simulink model "model"  (R2020a)
settings: Solver=VariableStepAuto  StartTime=0.0  StopTime=.3  MaxStep=1e-6  RelTol=1e-3  EnableMultiTasking=on
values from neighbouring files (symbols this model uses):
  f = 20    [data_collection.m]
  g = A(q,8)    [data_collection.m]
  g0 = 14e-6    (= 1.4e-05)    [data_collection.m]
  lf = 400e-6    (= 0.0004)    [data_collection.m]
  m = 2.0933e-6    (= 2.0933e-06)    [data_collection.m]
  tfd = 25e-6    (= 2.5e-05)    [data_collection.m]
  tp = 120e-9    (= 1.2e-07)    [data_collection.m]
  wb = 30e-6    (= 3e-05)    [data_collection.m]
  wt = 9e-6    (= 9e-06)    [data_collection.m]
libraries: simulink x1
settings Model: SimulationMode=accelerator  Creator=OXAALJ  LastModifiedBy=galarm2
settings SolverCC: MaxOrder=2  MaxConsecutiveZCs=10  MaxConsecutiveMinStep=10  ZeroCrossControl=DisableAll
settings DataIOCC: LimitDataPoints=on  SaveFormat=Array  DSMLogging=off  ReturnWorkspaceOutputs=off
settings OptimizationCC: EfficientMapNaN2IntZero=off  LifeSpan=inf
settings DebuggingCC: UnderspecifiedInitializationDetection=Classic  MergeDetectMultiDrivingBlocksExec=none  SolverPrmCheckMsg=warning  MultiTaskDSMMsg=warning  MultiTaskCondExecSysMsg=none  StateNameClashWarn=warning  SFUnexpectedBacktrackingDiag=warning  SFNoUnconditionalDefaultTransitionDiag=warning  SFExecutionAtInitializationDiag=none  ArithmeticOperatorsInVariantConditions=warning
settings HardwareCC: ProdBitPerPointer=32  ProdBitPerSizeT=32  ProdBitPerPtrDiffT=32  ProdLargestAtomicFloat=None  ProdIntDivRoundTo=Undefined  ProdEndianess=Unspecified  ProdWordSize=32  ProdHWDeviceType=32-bit Generic  TargetBitPerPointer=64  TargetBitPerSizeT=64  TargetBitPerPtrDiffT=64  TargetLongLongMode=on  TargetIntDivRoundTo=Zero  TargetEndianess=LittleEndian  TargetWordSize=64  TargetHWDeviceType=MATLAB Host  ProdEqTarget=off
settings ModelReferenceCC: PropagateSignalLabelsOutOfModel=off
settings SFSimCC: SimUseLocalCustomCode=off  CustomCodeUndefinedFunction=UseInterfaceOnly
settings CodeAppCC: MaxIdLength=128
settings GRTTargetCC: TargetLangStandard=C89/C90 (ANSI)  CombineOutputUpdateFcns=off  GRTInterface=on
settings ConfigComp: CovMetricSettings=dw  CovHtmlReporting=on  CovSaveCumulativeToWorkspaceVar=on  CovSaveSingleToWorkspaceVar=on  CovExternalEMLEnable=off  CovSFcnEnable=off

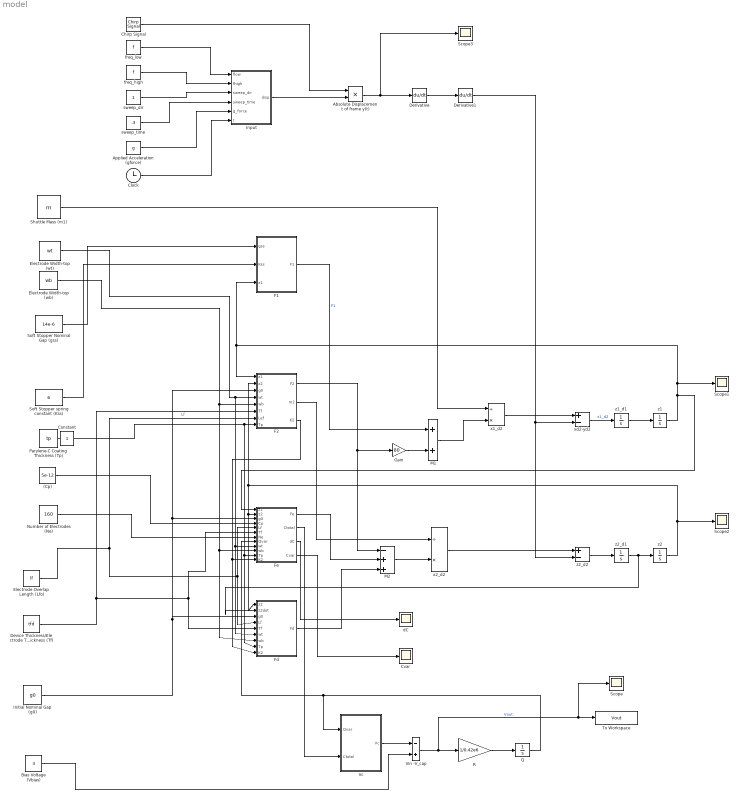
== system model ==
  " M2" : Sum  Inputs=-++  RndMeth=Nearest
  (Cp) : Constant  Value=5e-12  VectorParams1D=off
  Absolute Displacement of frame y(t) : Product
  Applied Acceleration (gforce) : Constant  Value=g
  Bias Voltage (Vbias) : Constant  Value=3
  Chirp Signal : simulink/Sources/Chirp Signal  f1=f  T=0.3  f2=f
  Clock : Clock
  Cvar : Scope
  Derivative : Derivative
  Derivative1 : Derivative
  Device Thickness/Electrode Thickness (Tf) : Constant  Value=tfd
  Electrode Overlap Length (Lfo) : Constant  Value=lf
  Electrode Width-top (wb) : Constant  Value=wb
  Electrode Width-top (wt) : Constant  Value=wt
  F1 : MATLAB Function  TreatAsAtomicUnit=on
  F2 : MATLAB Function  TreatAsAtomicUnit=on
  Fd : MATLAB Function  TreatAsAtomicUnit=on
  Fe : MATLAB Function  TreatAsAtomicUnit=on
  Gain : Gain  Gain=80
  Initial Nominal Gap (g0) : Constant  Value=g0
  Input : MATLAB Function  TreatAsAtomicUnit=on
  M1 : Sum  RndMeth=Nearest
  Number of Electrodes (Ne) : Constant  Value=160
  Parylene-C Coating Thickness (Tp) : Constant  Value=tp
  Q : Integrator
  R : Gain  Gain=1/0.42e6
  Scope{,1..3} (4 alike) : Scope
  Shuttle Mass (m1) : Constant  Value=m
  Soft Stopper Nominal Gap (gss) : Constant  Value=14e-6
  Soft Stopper spring constant (Kss) : Constant  Value=6
  To Workspace : ToWorkspace  VariableName=Vout  SampleTime=-1
      settings: Save2DSignal=2-D array (concatenate along first dimension)
  Vc : MATLAB Function  TreatAsAtomicUnit=on
  Vin -V_cap : Sum  Inputs=-+  RndMeth=Nearest
  dC : Scope
  freq_high : Constant  Value=f
  freq_low : Constant  Value=f
  sweep_dir : Constant
  sweep_time : Constant  Value=.3
  x1_d2 : Product  Inputs=/*
  x2_d2 : Product  Inputs=/*
  xd2-yd2 : Sum  Inputs=+-  RndMeth=Nearest
  z1 : Integrator
  z1_d1 : Integrator
  z2 : Integrator
  z2_d1 : Integrator
  z2_d2 : Sum  Inputs=+-  RndMeth=Nearest
  Constant : Constant  IOType=siggen
  wires:
  F1/1(F1) -> M1/1  "F1"
  Shuttle Mass (m1)/1 -> x1_d2/1
  Initial Nominal Gap (g0)/1 -> F2/3(g0), Fe/3(g0), Fd/3(g0)
  Bias Voltage (Vbias)/1 -> Vin -V_cap/2
  Vin -V_cap/1 -> Scope/1, To Workspace/1, R/1  "Vout"
  R/1 -> Q/1
  Q/1 -> Fe/8(Qvar), Vc/1(Qvar)
  Electrode Overlap Length (Lfo)/1 -> F2/7(Lef), Fd/4(Lf), Fe/5(Lf)  "Lf"
  (Cp)/1 -> Fe/4(Cp)
  Device Thickness/Electrode Thickness (Tf)/1 -> F2/6(Tf), Fd/5(Tf), Fe/6(Tf)
  Soft Stopper spring constant (Kss)/1 -> F1/2(Kss)
  M1/1 -> x1_d2/2
  x1_d2/1 -> xd2-yd2/1
  xd2-yd2/1 -> z1_d1/1  "z1_d2"
  z1_d1/1 -> z1/1
  x2_d2/1 -> z2_d2/1
  z2_d1/1 -> Fd/2(z2dot), z2/1
  z2/1 -> Scope2/1, Fd/1(z2), Fe/2(z2), F2/2(z2)
  " M2"/1 -> x2_d2/2
  Soft Stopper Nominal Gap (gss)/1 -> F1/1(gss)
  Input/1(disp) -> Absolute Displacement of frame y(t)/2
  freq_high/1 -> Input/2(fhigh)
  Applied Acceleration (gforce)/1 -> Input/5(g_force)
  Clock/1 -> Input/6(t)
  F2/1(F2) -> Gain/1, " M2"/1
  F2/2(m2) -> x2_d2/1
  Parylene-C Coating Thickness (Tp)/1 -> Fd/8(Tp), Fe/11(Tp), F2/8(Tp)
  Fe/1(Fe) -> " M2"/2
  Fe/2(Ctotal) -> Vc/2(Ctotal)
  Fd/1(Fd) -> " M2"/3
  Vc/1(Vc) -> Vin -V_cap/1
  Electrode Width-top (wt)/1 -> Fd/6(wt), Fe/9(wt), F2/4(wt)
  Electrode Width-top (wb)/1 -> Fd/7(wb), Fe/10(wb), F2/5(wb)
  Absolute Displacement of frame y(t)/1 -> Scope3/1, Derivative/1
  Derivative/1 -> Derivative1/1
  freq_low/1 -> Input/1(flow)
  sweep_time/1 -> Input/4(sweep_time)
  sweep_dir/1 -> Input/3(sweep_dir)
  z2_d2/1 -> z2_d1/1
  Derivative1/1 -> z2_d2/2, xd2-yd2/2
  Gain/1 -> M1/2
  z1/1 -> Scope1/1, F2/1(z1), F1/3(z1), Fe/1(z1)
  Number of Electrodes (Ne)/1 -> Fe/7(Ne)
  Fe/3(dC) -> dC/1
  Fe/4(Cvar) -> Cvar/1
  F2/3(K2) -> Fd/9(K2), Fe/12(K2)
  Chirp Signal/1 -> Absolute Displacement of frame y(t)/1

== matlab function model/F1 ==
  data: gss input; Kss input; z1 input; F1 output
function F1 = fcn(gss,Kss,z1)
% This function calculates the force F1
% Device Parameters

% Meg Value
k1 = 0.16;
Fsp = (-k1.*z1); % suspension beam force

% Fss
if abs(z1) < gss
    Fss = 0; % stopper not engaged
else
    Fss = Kss*(abs(z1)-gss)*sign(z1); % stopper is engaged
end

F1 = Fss + Fsp;
end

== matlab function model/Fd ==
  data: z2 input; z2dot input; g0 input; Fd output; Lf input; Tf input; wt input; wb input; Tp input; K2 input
function Fd = fcn(z2,z2dot,g0,Lf,Tf,wt,wb,Tp,K2)
% This function calculates the force F2
% Device Parameters
gp = g0 - 2*Tp; % minimum air gap 
eta = 1.849e-5; % Dynamic viscosity of air (kg/m*s)
% ws = mean([wt,wb]); % Avg. Electrode width
% I = (1/12)*Tf*(ws^3); % Moment of Inertia average width
% E = 180e9; % The Young's modulous 

% Scaling term for Damping force
scale = 0.015;
% set = 0;
% if abs(z2) >= gp
%     set = set + 1;
% end
% 
% if set < 1
%     scale = 0.015; % Scaling term for Damping force
% else
%     scale = 0.01965; 
% end

% Tilt angle
a = (wb-wt)/Lf; % previous calculation
% a = ((wb-wt)/Lf)-(((K2*(abs(z2)-gp))*(Lf^2))/(3*E*I)); % new calculation

% Fd_l
ul  =  gp + z2; % Left-hand side ho
ll  =  ul + a*Lf; % Left-hand side hl
A1_l  =  -ul*Lf/(ul + 2*a)* z2dot; % The c1 parameter, left
A2_l  =  12*eta*a^-2/(2*ul + a*Lf) * z2dot; % The c1 parameter, left
Fd_l   =  Tf*(Lf*A2_l - 6*eta*Lf/a/ul/ll*A1_l + 6*eta*Lf*a^-4/ll*z2dot + 12*eta*a^-3 * z2dot * (log(abs(ul./ll))) );

% Fd_r
ur  =  gp - z2;  
lr  =  ur + a*Lf;
A1_r  =  -ur*Lf/(ur + 2*a)* z2dot; % The c1 parameter, right
A2_r  =  12*eta*a^-2/(2*ur + a*Lf) * z2dot; % The c1 parameter, right
Fd_r   =  Tf*(Lf*A2_r - 6*eta*Lf/a/ur/lr*A1_r + 6*eta*Lf*a^-4/lr*z2dot - 12*eta*a^-3 * z2dot * (log(abs(ur./lr))) );

% Fd
Fd  =  -scale*(Fd_l + Fd_r);
end

== matlab function model/Vc ==
  data: Qvar input; Vc output; Ctotal input
function Vc = fcn(Qvar,Ctotal)
% This function calculates the Vc value
Vc = Qvar/Ctotal;
end

== matlab function model/Fe ==
  data: z1 input; z2 input; g0 input; Cp input; Fe output; Lf input; Tf input; Ne input; Qvar input; wt input; wb input; Tp input; Ctotal output; dC output; Cvar output; K2 input
function [Fe,Ctotal,dC,Cvar] = fcn(z1,z2,g0,Cp,Lf,Tf,Ne,Qvar,wt,wb,Tp,K2)
% This function calculates the force F2
% Device Parameters
gp = g0 - 2*Tp; % minimum air gap 
ws = mean([wt,wb]); % Avg. Electrode width
I = (1/12)*Tf*(ws^3); % Moment of Inertia average width
E = 180e9; % The Young's modulous 
e = 8.85e-12; % Permittivity of free space
ep = 3.2; % Relative Permittivity of Parylene-C
scale = 1;
Cvar = 0;

% Tilt angle
a = (wb-wt)/Lf; % previous calculation
% a = ((wb-wt)/Lf)-(((K2*(abs(z2)-g0))*(Lf^2))/(3*E*I)); % new calculation

if abs(z2) < gp % The electrodes are not in contact
    % Cvar_r
    Crl = (ep.*e.*Lf.*Tf)/Tp;
    Cair_r = ((e.*Tf)/(2.*a)).*(log(((g0 - z2 + 2.*a.*Lf)./(g0 - z2))));
    Cvar_r = 1/((1/Crl)+(1/Cair_r)+(1/Crl));
    % Cvar_l
    Cair_l = ((e.*Tf)./(2.*a)).*(log(((g0 + z2 + 2.*a.*Lf)./(g0 + z2))));
    Cvar_l = 1./((1/Crl)+(1/Cair_l)+(1/Crl));
    % Cvar
    Cvar = (Cvar_r + Cvar_l).*(Ne/2);
elseif abs(z2) >= gp % The electrodes are in contact
    % Colliding Electrode
    Crl = (ep.*e.*Lf.*Tf)/Tp;
    % d = (wb-wt)-(((K2*(abs(z1)-abs(z2))*(Lf^3))/(3*E*I)));
    % d = (wb-wt)-(((K2*(abs(z1)-g0)*(Lf^3))/(3*E*I)));
    d = (wb-wt)-(((K2*(abs(z2)-g0))*(Lf^3))/(3*E*I));
    % Cair_c = ((e*Tf*(Lf^2))/(2*d))*(log(abs(d-2*Tp))-log(abs((2*Tp))));
    % Cair_c = ((e*Tf*Lf)/(d))*(log((2*d - 2*Tp)/(2*Tp)));
    Cair_c = ((e*Tf*Lf)/(d))*(log((2*Tp + 2*d)/(2*Tp)));
    Cvar_c = 1./((1/Crl)+(1/Cair_c)+(1/Crl));
    % Non-colliding Electrode
    Cair_nc = ((e.*Tf)./(2.*a)).*(log((g0 + abs(z2) + 2.*a.*Lf)./(g0 + abs(z2))));
    Cvar_nc = 1./((1/Crl)+(1/Cair_nc)+(1/Crl));
    % Cvar
    Cvar = (Cvar_nc + Cvar_c).*(Ne/2);     
end

% Ctotal
Ctotal = Cvar + Cp;

% dC is divided by four here because nf is total electrodes, not number of electrode pairs
dC = ((e*Ne*Tf)./(4.*a))*( ((2*z2)/(gp^2 - z2^2)) - ((2*z2)/((gp + 2*Lf*a)^2 - z2^2) ));
% dC = ((e*Ne*Lf)./(4.*a))*( ((2*z2)/(g0^2 - z2^2)) - ((2*z2)/((g0 + 2*Tf*a)^2 - z2^2) ));

% dC = (Ne*((2*((g0 + 2*wb - 2*wt - z2)/(g0 - z2)^2 - 1/(g0 - z2))*(g0 - z2)*(wb - wt))/(Lf*Tf*e*log((g0 + 2*wb - 2*wt - z2)/(g0 - z2))^2*((2*wb - 2*wt)/(Lf*Tf*e*log((g0 + 2*wb - 2*wt - z2)/(g0 - z2))) + (2*Tp)/(Lf*Tf*e*ep))^2*(g0 + 2*wb - 2*wt - z2)) + (2*(g0 + z2)*(wb - wt)*(1/(g0 + z2) - (g0 + 2*wb - 2*wt + z2)/(g0 + z2)^2))/(Lf*Tf*e*log((g0 + 2*wb - 2*wt + z2)/(g0 + z2))^2*((2*wb - 2*wt)/(Lf*Tf*e*log((g0 + 2*wb - 2*wt + z2)/(g0 + z2))) + (2*Tp)/(Lf*Tf*e*ep))^2*(g0 + 2*wb - 2*wt + z2))))/2;
% dC = (Ne*(((K2*Lf^2*sign(z2))/(3*E*I*Tf*e*log(((2*K2*(g0 - abs(z2))*Lf^3)/(3*E*I) + 2*Tp + 2*wb - 2*wt)/(2*Tp))) - (2*K2*Lf^2*sign(z2)*((K2*(g0 - abs(z2))*Lf^3)/(3*E*I) + wb - wt))/(3*E*I*Tf*e*log((2*Tp + 2*wb - 2*wt + (2*K2*Lf^3*(g0 - abs(z2)))/(3*E*I))/(2*Tp))^2*((2*K2*(g0 - abs(z2))*Lf^3)/(3*E*I) + 2*Tp + 2*wb - 2*wt)))/((wb - wt + (K2*Lf^3*(g0 - abs(z2)))/(3*E*I))/(Lf*Tf*e*log((2*Tp + 2*wb - 2*wt + (2*K2*Lf^3*(g0 - abs(z2)))/(3*E*I))/(2*Tp))) + (2*Tp)/(Lf*Tf*e*ep))^2 + (2*(sign(z2)/(g0 + abs(z2)) - (sign(z2)*(g0 + 2*wb - 2*wt + abs(z2)))/(g0 + abs(z2))^2)*(g0 + abs(z2))*(wb - wt))/(Lf*Tf*e*log((g0 + 2*wb - 2*wt + abs(z2))/(g0 + abs(z2)))^2*((2*wb - 2*wt)/(Lf*Tf*e*log((g0 + 2*wb - 2*wt + abs(z2))/(g0 + abs(z2)))) + (2*Tp)/(Lf*Tf*e*ep))^2*(g0 + 2*wb - 2*wt + abs(z2)))))/2;

% dC = 0;
% % For no collision
% if abs(z2) < gp % The electrodes are not in contact
%     % g0
%     dC = (Ne*((2*((g0 + 2*wb - 2*wt - z2)/(g0 - z2)^2 - 1/(g0 - z2))*(g0 - z2)*(wb - wt))/(Lf*Tf*e*log((g0 + 2*wb - 2*wt - z2)/(g0 - z2))^2*((2*wb - 2*wt)/(Lf*Tf*e*log((g0 + 2*wb - 2*wt - z2)/(g0 - z2))) + (2*Tp)/(Lf*Tf*e*ep))^2*(g0 + 2*wb - 2*wt - z2)) + (2*(g0 + z2)*(wb - wt)*(1/(g0 + z2) - (g0 + 2*wb - 2*wt + z2)/(g0 + z2)^2))/(Lf*Tf*e*log((g0 + 2*wb - 2*wt + z2)/(g0 + z2))^2*((2*wb - 2*wt)/(Lf*Tf*e*log((g0 + 2*wb - 2*wt + z2)/(g0 + z2))) + (2*Tp)/(Lf*Tf*e*ep))^2*(g0 + 2*wb - 2*wt + z2))))/2;
%     % gp
%     % dC = (Ne*((2*((gp + 2*wb - 2*wt - z2)/(gp - z2)^2 - 1/(gp - z2))*(gp - z2)*(wb - wt))/(Lf*Tf*e*log((gp + 2*wb - 2*wt - z2)/(gp - z2))^2*((2*wb - 2*wt)/(Lf*Tf*e*log((gp + 2*wb - 2*wt - z2)/(gp - z2))) + (2*Tp)/(Lf*Tf*e*ep))^2*(gp + 2*wb - 2*wt - z2)) + (2*(gp + z2)*(wb - wt)*(1/(gp + z2) - (gp + 2*wb - 2*wt + z2)/(gp + z2)^2))/(Lf*Tf*e*log((gp + 2*wb - 2*wt + z2)/(gp + z2))^2*((2*wb - 2*wt)/(Lf*Tf*e*log((gp + 2*wb - 2*wt + z2)/(gp + z2))) + (2*Tp)/(Lf*Tf*e*ep))^2*(gp + 2*wb - 2*wt + z2))))/2;
% % For collision
% elseif abs(z2) >= gp % The electrodes are in contact
%     % g0
%     dC = (Ne*(((K2*Lf^2*sign(z2))/(3*E*I*Tf*e*log(((2*K2*(g0 - abs(z2))*Lf^3)/(3*E*I) + 2*Tp + 2*wb - 2*wt)/(2*Tp))) - (2*K2*Lf^2*sign(z2)*((K2*(g0 - abs(z2))*Lf^3)/(3*E*I) + wb - wt))/(3*E*I*Tf*e*log((2*Tp + 2*wb - 2*wt + (2*K2*Lf^3*(g0 - abs(z2)))/(3*E*I))/(2*Tp))^2*((2*K2*(g0 - abs(z2))*Lf^3)/(3*E*I) + 2*Tp + 2*wb - 2*wt)))/((wb - wt + (K2*Lf^3*(g0 - abs(z2)))/(3*E*I))/(Lf*Tf*e*log((2*Tp + 2*wb - 2*wt + (2*K2*Lf^3*(g0 - abs(z2)))/(3*E*I))/(2*Tp))) + (2*Tp)/(Lf*Tf*e*ep))^2 + (2*(sign(z2)/(g0 + abs(z2)) - (sign(z2)*(g0 + 2*wb - 2*wt + abs(z2)))/(g0 + abs(z2))^2)*(g0 + abs(z2))*(wb - wt))/(Lf*Tf*e*log((g0 + 2*wb - 2*wt + abs(z2))/(g0 + abs(z2)))^2*((2*wb - 2*wt)/(Lf*Tf*e*log((g0 + 2*wb - 2*wt + abs(z2))/(g0 + abs(z2)))) + (2*Tp)/(Lf*Tf*e*ep))^2*(g0 + 2*wb - 2*wt + abs(z2)))))/2;
%     % gp
%     % dC = (Ne*(((K2*Lf^2*sign(z2))/(3*E*I*Tf*e*log(((2*K2*(gp - abs(z2))*Lf^3)/(3*E*I) + 2*Tp + 2*wb - 2*wt)/(2*Tp))) - (2*K2*Lf^2*sign(z2)*((K2*(gp - abs(z2))*Lf^3)/(3*E*I) + wb - wt))/(3*E*I*Tf*e*log((2*Tp + 2*wb - 2*wt + (2*K2*Lf^3*(gp - abs(z2)))/(3*E*I))/(2*Tp))^2*((2*K2*(gp - abs(z2))*Lf^3)/(3*E*I) + 2*Tp + 2*wb - 2*wt)))/((wb - wt + (K2*Lf^3*(gp - abs(z2)))/(3*E*I))/(Lf*Tf*e*log((2*Tp + 2*wb - 2*wt + (2*K2*Lf^3*(gp - abs(z2)))/(3*E*I))/(2*Tp))) + (2*Tp)/(Lf*Tf*e*ep))^2 + (2*(sign(z2)/(gp + abs(z2)) - (sign(z2)*(gp + 2*wb - 2*wt + abs(z2)))/(gp + abs(z2))^2)*(gp + abs(z2))*(wb - wt))/(Lf*Tf*e*log((gp + 2*wb - 2*wt + abs(z2))/(gp + abs(z2)))^2*((2*wb - 2*wt)/(Lf*Tf*e*log((gp + 2*wb - 2*wt + abs(z2))/(gp + abs(z2)))) + (2*Tp)/(Lf*Tf*e*ep))^2*(gp + 2*wb - 2*wt + abs(z2)))))/2;
% end

% Fe
NFe = -1*((Qvar^2)/(2*Ctotal^2))*dC;
Fe = NFe./(Ne/2)*scale;
end

== matlab function model/Input ==
  data: flow input; fhigh input; sweep_dir input; sweep_time input; g_force input; disp output; t input
function disp  = fcn(flow,fhigh,sweep_dir,sweep_time,g_force,t)
ramp = 200e-3;

if sweep_dir > 0
    %upsweep
    if t < ramp
        freq = (t/sweep_time)*(fhigh-flow) + flow;
        disp = (t/ramp)* (g_force/(4.0243*freq^2)); %const = (2*pi())^2/9.81
        % vel = (t/ramp)*(g_force*9.81)/(2*pi*freq);
    else
        freq = (t/sweep_time)*(fhigh-flow) + flow;
        disp = g_force/(4.0243*freq^2);   %const = (2*pi())^2/9.81
        % vel = (g_force*9.81)/(2*pi*freq);
        % disp = g/(4.0243*((fhigh-flow)/2)^2); 
        % freq = (0.5) * (fhigh+flow);
        % disp = g/(4.0243*freq^2);  %const = (2*pi())^2/9.81
    end
else
    %downsweep
    if t < ramp
        freq = fhigh - (t/sweep_time)*(fhigh-flow);
        disp = (t/ramp)* (g_force/(4.0243*freq^2)); %const = (2*pi())^2/9.81
        % vel = (t/ramp)*(g_force*9.81)/(2*pi*freq);
    else
        freq = fhigh - (t/sweep_time)*(fhigh-flow);
        disp = g_force/(4.0243*freq^2);  %const = (2*pi())^2/9.81
        % vel = (g_force*9.81)/(2*pi*freq);
        % disp = g/(4.0243*((fhigh-flow)/2)^2); 
        % freq = (0.5) * (fhigh+flow);
        % disp = g/(4.0243*freq^2);  %const = (2*pi())^2/9.81
    end
end
end

== matlab function model/F2 ==
  data: z1 input; z2 input; F2 output; g0 input; m2 output; wt input; wb input; Tf input; Lef input; Tp input; K2 output
function [F2,m2,K2] = fcn(z1,z2,g0,wt,wb,Tf,Lef,Tp)
% This function calculates the force F2
% Device Parameters
gp = g0 - 2*Tp; % minimum air gap
E = 180e9; % The Young's modulous 
rho = 2333; % density (kg/m3)
ws = mean([wt,wb]); % Avg. Electrode width
Lf = Lef + 50e-6; % Account for non-overlap
I = (1/12)*Tf*(ws^3); % Moment of Inertia average width
% h = (wb-wt)*(Lef/Lf); % height function
% I = (1/12)*Tf*(h^3); % Moment of Inertia height function

% NF2 and Nm2
if abs(z2) < gp
    m2 = (33/140)*rho*Tf*Lf*ws; % Mass of single electrode
    K2 = (1/4)*E/Lf^3*I; % Spring constant of electrode
    % K2 = 135801;
    F2 = -K2*(z1-z2);
  
else    
    m2 = 2*(33/140)*rho*Tf*Lf*ws; % Mass of combined electrode
    K2 = (1/4)*E/Lf^3*I; % Spring constant of electrode
    % K2 = 135801;
    % F2 = -K2*(z1-z2);
    F2 = -K2*(z1-z2) + K2*(abs(z2)-gp)*sign(z2);
end
end
